simulink model "Atos_Simulink15.3.19"  (R2018b)
settings: Solver=VariableStepAuto  StartTime=0  StopTime=24  FixedStep=1  RelTol=1.0e-3  AbsTol=1.0e-3  EnableMultiTasking=on
libraries: fl_lib x33, nesl_utility x15, SimscapeFluids_lib x2
settings Model: Creator=psytg1  LastModifiedBy=shama
settings SolverCC: AutoScaleAbsTol=off  MaxConsecutiveMinStep=50
settings DataIOCC: LimitDataPoints=on  MaxDataPoints=10000
settings OptimizationCC: LifeSpan=inf
settings DebuggingCC: AllowSymbolicDim=off  LibraryContextMissingDiagnostic=none  SFUnexpectedBacktrackingDiag=warning  SFNoUnconditionalDefaultTransitionDiag=warning  SFExecutionAtInitializationDiag=none
settings SFSimCC: SimUseLocalCustomCode=off
settings RTWCC: GenCodeOnly=on  RTWUseLocalCustomCode=off  TargetLang=C++
settings CodeAppCC: StateflowObjectComments=on
settings GRTTargetCC: TargetLangStandard=C++03 (ISO)  GeneratePreprocessorConditionals=Disable all  MultiInstanceERTCode=on  CodeInterfacePackaging=C++ class
settings ConfigComp: CovMetricSettings=dw  CovHtmlReporting=on  CovSaveCumulativeToWorkspaceVar=on  CovSaveSingleToWorkspaceVar=on  CovExternalEMLEnable=off  CovSFcnEnable=off
settings SimscapeCC: ExplicitSolverDiagnosticOptions=none  SimscapeLogType=all  SimscapeLogDataHistory=10000

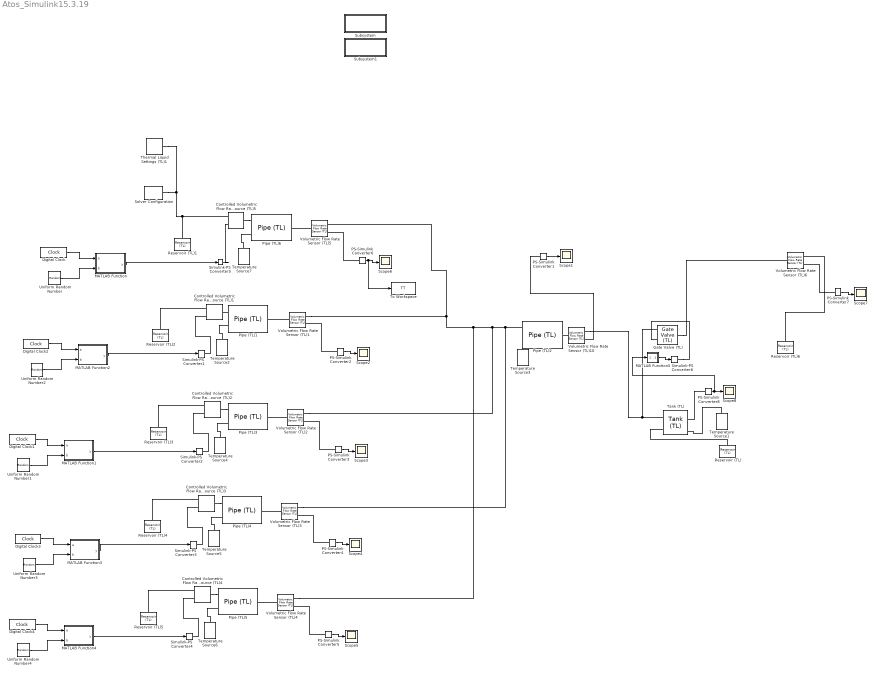
== system Atos_Simulink15.3.19 ==
  Controlled Volumetric Flow Rate Source (TL){1..5} (5 alike) : fl_lib/Thermal Liquid/Sources/Controlled Volumetric Flow Rate Source (TL)  area=3.14 m^2  length=0.1 m  mdot_A_specify=off  mdot_A_priority=None  mdot_A=1 kg/s  mdot_A_nominal_specify=off  mdot_A_nominal_unit=kg/s  mdot_A_nominal_value=1
      settings: SourceProductName=Simscape  SourceProductBaseCode=SS
  Digital Clock{,1..4} (5 alike) : DigitalClock
  Gate Valve (TL) : SimscapeFluids_lib/Thermal Liquid/Valves & Orifices/Flow Control Valves/Gate Valve (TL)  diam_orifice=3 m  x_0=0 m  area_leak=1e-12 m^2  smoothing_factor=1  area=30 m^2  length=1 m  Cd=0.7  Re_c=12  mdot_A_specify=off  mdot_A_priority=None  mdot_A=1 kg/s  mdot_A_nominal_specify=off  mdot_A_nominal_unit=kg/s  mdot_A_nominal_value=1
      settings: SourceProductName=Simscape Fluids  SourceProductBaseCode=SH
  MATLAB Function : MATLAB Function  TreatAsAtomicUnit=on
  MATLAB Function1 : MATLAB Function  TreatAsAtomicUnit=on
  MATLAB Function2 : MATLAB Function  TreatAsAtomicUnit=on
  MATLAB Function3 : MATLAB Function  TreatAsAtomicUnit=on
  MATLAB Function4 : MATLAB Function  TreatAsAtomicUnit=on
  MATLAB Function5 : MATLAB Function  TreatAsAtomicUnit=on
  PS-Simulink Converter{1..8} (8 alike) : nesl_utility/PS-Simulink Converter  PhysicalDomain=network_engine_domain  SubClassName=ps_output  LeftPortType=input  RightPortType=output  PseudoPeriodic=off  Frequencies=[]  Unit=1  AffineConversion=off
  Pipe (TL){1,3..6} (5 alike) : fl_lib/Thermal Liquid/Elements/Pipe (TL)  dynamic_compressibility=1  inertia=0  length=5 m  area=CrossArea m^2  Dh=0.1128 m  length_add=1 m  roughness=15e-6 m  Re_lam=2000  Re_tur=4000  shape_factor=64  Nu_lam=3.66  p0=0.101325 MPa  T0=281.15 K  mdot0=0 kg/s
      settings: SourceProductName=Simscape  SourceProductBaseCode=SS
  Pipe (TL)2 : fl_lib/Thermal Liquid/Elements/Pipe (TL)  dynamic_compressibility=1  inertia=0  length=10 m  area=30 m^2  Dh=0.1128 m  length_add=1 m  roughness=15e-6 m  Re_lam=2000  Re_tur=4000  shape_factor=64  Nu_lam=3.66  p0=0.101325 MPa  T0=281.15 K  mdot0=0 kg/s
      settings: SourceProductName=Simscape  SourceProductBaseCode=SS
  Reservoir (TL) : fl_lib/Thermal Liquid/Elements/Reservoir (TL)  pressure_spec=1  reservoir_pressure=0.101325 MPa  reservoir_temperature=293.15 K  area=3.14 m^2
      settings: SourceProductName=Simscape  SourceProductBaseCode=SS
  Reservoir (TL){1..5} (5 alike) : fl_lib/Thermal Liquid/Elements/Reservoir (TL)  pressure_spec=1  reservoir_pressure=0.101325 MPa  reservoir_temperature=293.15 K  area=0.01 m^2
      settings: SourceProductName=Simscape  SourceProductBaseCode=SS
  Reservoir (TL)6 : fl_lib/Thermal Liquid/Elements/Reservoir (TL)  pressure_spec=1  reservoir_pressure=0.101325 MPa  reservoir_temperature=293.15 K  area=15.7 m^2
      settings: SourceProductName=Simscape  SourceProductBaseCode=SS
  Scope{1..8} (8 alike) : Scope
  Simulink-PS Converter{1..6} (6 alike) : nesl_utility/Simulink-PS Converter  PhysicalDomain=network_engine_domain  SubClassName=ps_input  LeftPortType=input  RightPortType=output  PseudoPeriodic=off  Frequencies=[]  NoiseDistribution=none  NoiseParameters=[]  Unit=1  AffineConversion=off  FilteringAndDerivatives=filter  SimscapeFilterOrder=1  InputFilterTimeConstant=0.001  UdotUserProvided=0
  Solver Configuration : nesl_utility/Solver Configuration  PhysicalDomain=network_engine_domain  SubClassName=solver  LeftPortType=input  RightPortType=generic  Tones=[]  Harmonics=[]  SimulateNoise=off  Profile=off  UseLocalSampling=off  EnableSwitchedLinearOptims=on  FrequencyDomain=off  UseCCode=off  RelTol=0.001  AbsTol=1e-06  MinStep=1e-09  ToWorkspace=off  RevertToSquareIcSolve=off  NumHomotopyIterations=100  PhasorMode=off  PhasorModeNumHarmonics=1  DoDC=off  ResidualTolerance=1e-09  UseLocalSolver=off  LocalSolverChoice=NE_BACKWARD_EULER_ADVANCER  LocalSolverSampleTime=0.001  DoFixedCost=off  MaxNonlinIter=3  MaxModeIter=2  LinearAlgebra=Sparse  EquationFormulation=NE_TIME_EF  DelaysMemoryBudget=1024  AutomaticFiltering=on  FilteringTimeConstant=0.001  PartitionStorageMethod=AS_NEEDED  PartitionMemoryBudget=1024
  Subsystem : Subsystem
      settings: OpenFcn=open_system('simscape')
      mask Display: disp(sprintf('Open Simscape\nLibrary'));
  Subsystem1 : Subsystem
      settings: OpenFcn=|
      | load_system('fl_lib');
      | open_system('fl_lib/Thermal Liquid');
      mask Display: disp(sprintf('Open Thermal Liquid\nLibrary'));
  Tank (TL) : SimscapeFluids_lib/Thermal Liquid/Tanks & Accumulators/Tank (TL)  pressure_spec=1  tank_pressure=0.101325 MPa  max_capacity=10000 m^3  volume_spec=1  tank_area=50 m^2  level_TLU=[0, 3, 5] m  volume_TLU=[0, 4, 6] m^3  inlet_height=1 m  inlet_area=3.14 m^2  g=9.81 m/s^2  level_specify=on  level_priority=High  level=10 m  level_nominal_specify=off  level_nominal_unit=m  level_nominal_value=1  volume_specify=on  volume_priority=None  volume=10 m^3  volume_nominal_specify=off  volume_nominal_unit=m^3  volume_nominal_value=1  mass_specify=on  mass_priority=None  mass=10e+3 kg  mass_nominal_specify=off  mass_nominal_unit=kg  mass_nominal_value=1  T_tank_specify=on  T_tank_priority=High  T_tank=281.15 K  T_tank_nominal_specify=off  T_tank_nominal_unit=K  T_tank_nominal_value=1  inlet_heights_AB=[5, 1] m  inlet_areas_AB=[10, 1] m^2  inlet_heights_ABC=[5, 5, 1] m  inlet_areas_ABC=[10, 10, 1] m^2
      settings: SourceProductName=Simscape Fluids  SourceProductBaseCode=SH
  Temperature Source{1..7} (7 alike) : fl_lib/Thermal/Thermal Sources/Temperature Source  temperature=281.15 K
      settings: SourceProductName=Simscape
  Thermal Liquid Settings (TL)1 : fl_lib/Thermal Liquid/Utilities/Thermal Liquid Settings (TL)  table_dimensions=0  T_TLU=[273.1600 : 10 : 373.16]' K  p_TLU=[0.01, 0.1, 5 : 5 : 50] MPa  p_atm=0.101325 MPa  pT_region_flag=0  T_min=273.16 K  T_max=363.16 K  p_min=0.05 MPa  p_max=50 MPa  T_min_1D=273.16 K  T_max_1D=363.16 K  p_min_1D=0.05 MPa  p_max_1D=50 MPa  pT_validity_TLU=[1, 1, 1, 1, 1, 1, 1, 1, 1, 1, 1, 1; 1, 1, 1, 1, 1, 1, 1, 1, 1, 1, 1, 1; 1, 1, 1, 1, 1, 1, 1, 1, 1, 1, 1, 1; 1, 1, 1, 1, 1, 1, 1, 1, 1, 1, 1, 1; 1, 1, 1, 1, 1, 1, 1, 1, 1, 1, 1, 1; 0, 1, 1, 1, 1, 1, 1, 1, 1, 1, 1, 1; 0, 1, 1, 1, 1, 1, 1, 1, 1, 1, 1, 1; 0, 1, 1, 1, 1, 1, 1, 1, 1, 1, 1, 1; 0, 1, 1, 1, 1, 1, 1, 1, 1, 1, 1, 1; 0, 1, 1, 1, 1, 1, 1, 1, 1, 1, 1, 1; 0, 0, 1, 1, 1, 1, 1, 1, 1, 1, 1, 1]  rho_parameterization_2D=3  rho_parameterization_1D=1  rho_TLU=[999.7973, 999.8431, 1002.3216, 1004.8218, 1007.293, 1009.7358, 1012.1506, 1014.5379, 1016.8979, 1019.2311, 1021.538, 1023.8188; 999.6579, 999.7009, 1002.0303, 1004.382, 1006.7084, 1009.0101, 1011.2874, 1013.5407, 1015.7703, 1017.9766, 1020.1599, 1022.3206; 998.1632, 998.2045, 1000.4375, 1002.6924, 1004.9239, 1007.1324, 1009.3183, 1011.4819, 1013.6236, 1015.7438, 1017.8428, 1019.921; 995.6057, 995.6458, 997.81864, 1000.0128, 1002.1841, 1004.3332, 1006.4603, 1008.566, 1010.6505, 1012.7144, 1014.758, 1016.7815; 992.1724, 992.2119, 994.35133, 996.5113, 998.6484, 1000.7633, 1002.8563, 1004.928, 1006.9788, 1009.009, 1011.0192, 1013.0097; 988.02, 988.0299, 990.15684, 992.3035, 994.4268, 996.5273, 998.6056, 1000.6622, 1002.6976, 1004.7123, 1006.7067, 1008.6813; 983.18, 983.1901, 985.3217, 987.4721, 989.5983, 991.7008, 993.7803, 995.8374, 997.8726, 999.8864, 1001.8795, 1003.8522; 977.75, 977.7583, 979.9094, 982.0783, 984.2216, 986.34, 988.4343, 990.505, 992.5529, 994.5786, 996.5825, 998.5654; 971.77, 971.7836, 973.96734, 976.1678, 978.3409, 980.4876, 982.6087, 984.7049, 986.7768, 988.8254, 990.8511, 992.8545; 965.26, 965.3023, 967.53107, 969.7753, 971.9901, 974.1764, 976.3354, 978.4676, 980.5741, 982.6556, 984.7129, 986.7465; 958.62, 958.6315, 960.627, 962.9267, 965.1944, 967.4314, 969.6387, 971.8173, 973.9681, 976.0921, 978.19, 980.2628] kg/m^3  beta_TLU=[1.9649, 1.9654, 1.9929, 2.0213, 2.0499, 2.0787, 2.1078, 2.1372, 2.1668, 2.1966, 2.2268, 2.2572; 2.0913, 2.0918, 2.1191, 2.1471, 2.1752, 2.2036, 2.2322, 2.261, 2.2899, 2.3191, 2.3485, 2.3781; 2.1786, 2.1791, 2.2067, 2.235, 2.2634, 2.2919, 2.3206, 2.3494, 2.3784, 2.4075, 2.4367, 2.4661; 2.2332, 2.2337, 2.2619, 2.2908, 2.3197, 2.3487, 2.3778, 2.407, 2.4363, 2.4657, 2.4951, 2.5246; 2.26, 2.2605, 2.2895, 2.3191, 2.3487, 2.3784, 2.4081, 2.4378, 2.4675, 2.4973, 2.5272, 2.5571; 2.2638, 2.2638, 2.2936, 2.324, 2.3544, 2.3848, 2.4151, 2.4455, 2.4758, 2.5062, 2.5365, 2.5669; 2.2472, 2.2472, 2.2779, 2.3092, 2.3403, 2.3715, 2.4025, 2.4336, 2.4646, 2.4955, 2.5264, 2.5573; 2.214, 2.214, 2.2455, 2.2776, 2.3096, 2.3415, 2.3733, 2.405, 2.4367, 2.4683, 2.4998, 2.5313; 2.1668, 2.1668, 2.1992, 2.2321, 2.2649, 2.2976, 2.3301, 2.3626, 2.3949, 2.4272, 2.4593, 2.4914; 2.1081, 2.1081, 2.1413, 2.175, 2.2086, 2.2421, 2.2754, 2.3085, 2.3415, 2.3744, 2.4072, 2.4399; 2.0494, 2.0494, 2.0739, 2.1084, 2.1428, 2.177, 2.211, 2.2449, 2.2786, 2.3121, 2.3455, 2.3788] GPa  alpha_TLU=1e-4 * [-.679, -.676, -.49, -.307, -.13, .041, .206, .365, .519, .668, .811, .949; .878, .881, .998, 1.114, 1.227, 1.337, 1.445, 1.549, 1.651, 1.75, 1.846, 1.939; 2.068, 2.069, 2.141, 2.213, 2.283, 2.352, 2.42, 2.486, 2.551, 2.614, 2.676, 2.736; 3.034, 3.035, 3.074, 3.113, 3.152, 3.191, 3.229, 3.267, 3.305, 3.341, 3.377, 3.413; 3.855, 3.856, 3.87, 3.884, 3.899, 3.914, 3.93, 3.946, 3.961, 3.977, 3.993, 4.009; 4.578, 4.578, 4.572, 4.566, 4.562, 4.558, 4.555, 4.552, 4.55, 4.549, 4.548, 4.547; 5.233, 5.233, 5.209, 5.186, 5.165, 5.144, 5.125, 5.107, 5.09, 5.074, 5.059, 5.045; 5.84, 5.84, 5.801, 5.762, 5.725, 5.691, 5.657, 5.625, 5.595, 5.566, 5.538, 5.512; 6.414, 6.414, 6.36, 6.307, 6.256, 6.208, 6.161, 6.117, 6.074, 6.033, 5.994, 5.956; 6.967, 6.967, 6.898, 6.831, 6.766, 6.705, 6.646, 6.589, 6.535, 6.482, 6.432, 6.384; 7.519, 7.519, 7.423, 7.342, 7.264, 7.189, 7.118, 7.049, 6.983, 6.92, 6.859, 6.8] 1/K  rho_TLU_2=[999.7973, 999.8431, 1002.3216, 1004.8218, 1007.293, 1009.7358, 1012.1506, 1014.5379, 1016.8979, 1019.2311, 1021.538, 1023.8188; 999.6579, 999.7009, 1002.0303, 1004.382, 1006.7084, 1009.0101, 1011.2874, 1013.5407, 1015.7703, 1017.9766, 1020.1599, 1022.3206; 998.1632, 998.2045, 1000.4375, 1002.6924, 1004.9239, 1007.1324, 1009.3183, 1011.4819, 1013.6236, 1015.7438, 1017.8428, 1019.921; 995.6057, 995.6458, 997.81864, 1000.0128, 1002.1841, 1004.3332, 1006.4603, 1008.566, 1010.6505, 1012.7144, 1014.758, 1016.7815; 992.1724, 992.2119, 994.35133, 996.5113, 998.6484, 1000.7633, 1002.8563, 1004.928, 1006.9788, 1009.009, 1011.0192, 1013.0097; 988.02, 988.0299, 990.15684, 992.3035, 994.4268, 996.5273, 998.6056, 1000.6622, 1002.6976, 1004.7123, 1006.7067, 1008.6813; 983.18, 983.1901, 985.3217, 987.4721, 989.5983, 991.7008, 993.7803, 995.8374, 997.8726, 999.8864, 1001.8795, 1003.8522; 977.75, 977.7583, 979.9094, 982.0783, 984.2216, 986.34, 988.4343, 990.505, 992.5529, 994.5786, 996.5825, 998.5654; 971.77, 971.7836, 973.96734, 976.1678, 978.3409, 980.4876, 982.6087, 984.7049, 986.7768, 988.8254, 990.8511, 992.8545; 965.26, 965.3023, 967.53107, 969.7753, 971.9901, 974.1764, 976.3354, 978.4676, 980.5741, 982.6556, 984.7129, 986.7465; 958.62, 958.6315, 960.627, 962.9267, 965.1944, 967.4314, 969.6387, 971.8173, 973.9681, 976.0921, 978.19, 980.2628] kg/m^3  rho_ref_3=978.19 kg/m^3  T_ref_3=293.16 K  p_ref_3=0.101325 MPa  beta_const_3=2.1791 GPa  alpha_const_3=2.0691e-4 1/K  rho_TLU_4=[999.84; 999.7; 998.2; 995.65; 992.21; 988.03; 983.19; 977.76; 971.78; 965.3; 958.8] kg/m^3  beta_const_4=2.1791 GPa  p_ref_4=0.101325 MPa  rho_ref_5=998.21 kg/m^3  T_ref_5=293.16 K  p_ref_5=0.101325 MPa  beta_const_5=2.1791 GPa  alpha_const_5=2.0691e-4 1/K  u_parameterization_2D=1  u_parameterization_1D=1  u_TLU=[.0002, .0018, .086, .1588, .219, .267, .3034, .3288, .3436, .3483, .3435, .3294; 42.062, 42.06, 41.935, 41.804, 41.668, 41.527, 41.382, 41.233, 41.081, 40.924, 40.763, 40.599; 83.953, 83.948, 83.651, 83.349, 83.049, 82.749, 82.451, 82.153, 81.856, 81.56, 81.265, 80.971; 125.77, 125.76, 125.31, 124.86, 124.41, 123.97, 123.53, 123.1, 122.68, 122.25, 121.84, 121.42; 167.57, 167.56, 166.96, 166.37, 165.79, 165.21, 164.65, 164.09, 163.54, 163, 162.46, 161.94; 209.36, 209.36, 208.63, 207.9, 207.19, 206.48, 205.79, 205.11, 204.45, 203.79, 203.14, 202.5; 251.19, 251.19, 250.33, 249.47, 248.62, 247.79, 246.98, 246.18, 245.39, 244.62, 243.86, 243.12; 293.06, 293.06, 292.07, 291.07, 290.1, 289.14, 288.2, 287.28, 286.38, 285.49, 284.62, 283.77; 334.99, 334.99, 333.86, 332.73, 331.63, 330.54, 329.48, 328.44, 327.41, 326.41, 325.43, 324.46; 377, 377, 375.73, 374.46, 373.22, 372, 370.81, 369.64, 368.5, 367.38, 366.27, 365.19; 419.01, 419.01, 417.69, 416.27, 414.89, 413.54, 412.21, 410.91, 409.64, 408.4, 407.17, 405.98] kJ/kg  cp_TLU=[4.2199, 4.2194, 4.1957, 4.1726, 4.1508, 4.13, 4.1103, 4.0916, 4.0738, 4.0569, 4.0408, 4.0254; 4.1955, 4.1951, 4.1769, 4.1592, 4.1422, 4.1259, 4.1103, 4.0954, 4.0812, 4.0676, 4.0545, 4.0421; 4.1843, 4.184, 4.169, 4.1543, 4.1401, 4.1264, 4.1133, 4.1007, 4.0885, 4.0768, 4.0656, 4.0548; 4.1801, 4.1798, 4.1667, 4.1538, 4.1413, 4.1293, 4.1177, 4.1064, 4.0956, 4.0851, 4.075, 4.0653; 4.1796, 4.1794, 4.1675, 4.1558, 4.1444, 4.1334, 4.1227, 4.1123, 4.1023, 4.0926, 4.0832, 4.0741; 4.1813, 4.1813, 4.1702, 4.1592, 4.1484, 4.138, 4.1279, 4.1181, 4.1086, 4.0993, 4.0903, 4.0816; 4.185, 4.185, 4.1742, 4.1636, 4.1532, 4.1432, 4.1334, 4.1239, 4.1146, 4.1056, 4.0969, 4.0884; 4.1901, 4.1901, 4.1795, 4.169, 4.1588, 4.1489, 4.1393, 4.1299, 4.1207, 4.1118, 4.1032, 4.0947; 4.1968, 4.1968, 4.1862, 4.1757, 4.1655, 4.1555, 4.1458, 4.1364, 4.1273, 4.1183, 4.1096, 4.1012; 4.2052, 4.2052, 4.1944, 4.1837, 4.1733, 4.1632, 4.1534, 4.1438, 4.1345, 4.1255, 4.1166, 4.108; 4.2136, 4.2136, 4.2045, 4.1935, 4.1828, 4.1724, 4.1623, 4.1524, 4.1429, 4.1335, 4.1245, 4.1157] kJ/kg/K  u_TLU_2=[.0002, .0018, .086, .1588, .219, .267, .3034, .3288, .3436, .3483, .3435, .3294; 42.062, 42.06, 41.935, 41.804, 41.668, 41.527, 41.382, 41.233, 41.081, 40.924, 40.763, 40.599; 83.953, 83.948, 83.651, 83.349, 83.049, 82.749, 82.451, 82.153, 81.856, 81.56, 81.265, 80.971; 125.77, 125.76, 125.31, 124.86, 124.41, 123.97, 123.53, 123.1, 122.68, 122.25, 121.84, 121.42; 167.57, 167.56, 166.96, 166.37, 165.79, 165.21, 164.65, 164.09, 163.54, 163, 162.46, 161.94; 209.36, 209.36, 208.63, 207.9, 207.19, 206.48, 205.79, 205.11, 204.45, 203.79, 203.14, 202.5; 251.19, 251.19, 250.33, 249.47, 248.62, 247.79, 246.98, 246.18, 245.39, 244.62, 243.86, 243.12; 293.06, 293.06, 292.07, 291.07, 290.1, 289.14, 288.2, 287.28, 286.38, 285.49, 284.62, 283.77; 334.99, 334.99, 333.86, 332.73, 331.63, 330.54, 329.48, 328.44, 327.41, 326.41, 325.43, 324.46; 377, 377, 375.73, 374.46, 373.22, 372, 370.81, 369.64, 368.5, 367.38, 366.27, 365.19; 419.01, 419.01, 417.69, 416.27, 414.89, 413.54, 412.21, 410.91, 409.64, 408.4, 407.17, 405.98] kJ/kg  cp_TLU_3=[4.2199, 4.2194, 4.1957, 4.1726, 4.1508, 4.13, 4.1103, 4.0916, 4.0738, 4.0569, 4.0408, 4.0254; 4.1955, 4.1951, 4.1769, 4.1592, 4.1422, 4.1259, 4.1103, 4.0954, 4.0812, 4.0676, 4.0545, 4.0421; 4.1843, 4.184, 4.169, 4.1543, 4.1401, 4.1264, 4.1133, 4.1007, 4.0885, 4.0768, 4.0656, 4.0548; 4.1801, 4.1798, 4.1667, 4.1538, 4.1413, 4.1293, 4.1177, 4.1064, 4.0956, 4.0851, 4.075, 4.0653; 4.1796, 4.1794, 4.1675, 4.1558, 4.1444, 4.1334, 4.1227, 4.1123, 4.1023, 4.0926, 4.0832, 4.0741; 4.1813, 4.1813, 4.1702, 4.1592, 4.1484, 4.138, 4.1279, 4.1181, 4.1086, 4.0993, 4.0903, 4.0816; 4.185, 4.185, 4.1742, 4.1636, 4.1532, 4.1432, 4.1334, 4.1239, 4.1146, 4.1056, 4.0969, 4.0884; 4.1901, 4.1901, 4.1795, 4.169, 4.1588, 4.1489, 4.1393, 4.1299, 4.1207, 4.1118, 4.1032, 4.0947; 4.1968, 4.1968, 4.1862, 4.1757, 4.1655, 4.1555, 4.1458, 4.1364, 4.1273, 4.1183, 4.1096, 4.1012; 4.2052, 4.2052, 4.1944, 4.1837, 4.1733, 4.1632, 4.1534, 4.1438, 4.1345, 4.1255, 4.1166, 4.108; 4.2136, 4.2136, 4.2045, 4.1935, 4.1828, 4.1724, 4.1623, 4.1524, 4.1429, 4.1335, 4.1245, 4.1157] kJ/kg/K  u_TLU_4=[.0018; 42.06; 83.948; 125.76; 167.56; 209.36; 251.19; 293.06; 334.99; 377; 418.01] kJ/kg  cp_TLU_5=[4.2199; 4.1955; 4.1843; 4.1801; 4.1796; 4.1813; 4.185; 4.1901; 4.1968; 4.2052; 4.2136] kJ/kg/K  nu_TLU=[1.7917, 1.7914, 1.7763, 1.7615, 1.7473, 1.7338, 1.7208, 1.7085, 1.6967, 1.6854, 1.6747, 1.6645; 1.3061, 1.3059, 1.2986, 1.2914, 1.2845, 1.2779, 1.2716, 1.2656, 1.2598, 1.2543, 1.2491, 1.2441; 1.0032, 1.0032, .9995, .9959, .9924, .9891, .9859, .9829, .9801, .9774, .9748, .9724; .8006, .8005, .7987, .797, .7953, .7937, .7922, .7908, .7894, .7881, .787, .7859; .6577, .6577, .657, .6562, .6555, .6548, .6543, .6537, .6532, .6528, .6523, .652; .553, .553, .5529, .5527, .5526, .5525, .5524, .5524, .5524, .5524, .5524, .5525; .4739, .4739, .4741, .4743, .4745, .4747, .475, .4753, .4755, .4758, .4762, .4765; .4127, .4127, .4131, .4135, .4139, .4143, .4148, .4152, .4157, .4162, .4167, .4172; .3643, .3643, .3648, .3654, .3659, .3665, .367, .3676, .3682, .3688, .3694, .37; .3254, .3254, .3261, .3267, .3273, .328, .3286, .3293, .3299, .3306, .3312, .3319; .2866, .2866, .2945, .2952, .2959, .2965, .2972, .2979, .2986, .2993, .3, .3007] mm^2/s  nu_TLU_2=[1.7917; 1.3061; 1.0032; .8006; .6577; .553; .4739; .4127; .3643; .3254; .2866] mm^2/s  k_TLU=[561.04, 561.09, 563.8, 566.56, 569.32, 572.08, 574.82, 577.54, 580.24, 582.92, 585.57, 588.18; 580.02, 580.07, 582.45, 584.88, 587.32, 589.75, 592.18, 594.61, 597.02, 599.42, 601.8, 604.16; 598.44, 598.48, 600.73, 603.03, 605.33, 607.64, 609.94, 612.24, 614.54, 616.82, 619.1, 621.36; 615.48, 615.52, 617.73, 620, 622.26, 624.54, 626.81, 629.07, 631.34, 633.6, 635.85, 638.09; 630.6, 630.64, 632.87, 635.15, 637.44, 639.72, 642.01, 644.29, 646.57, 648.84, 651.11, 653.36; 643.61, 643.61, 645.88, 648.21, 650.53, 652.86, 655.18, 657.51, 659.82, 662.14, 664.44, 666.74; 654.39, 654.39, 656.73, 659.12, 661.5, 663.89, 666.27, 668.65, 671.02, 673.38, 675.74, 678.09; 663.13, 663.13, 665.54, 668, 670.46, 672.91, 675.36, 677.8, 680.24, 682.67, 685.09, 687.5; 670.02, 670.02, 672.51, 675.05, 677.59, 680.12, 682.64, 685.16, 687.67, 690.17, 692.66, 695.14; 675.27, 675.27, 677.85, 680.48, 683.11, 685.73, 688.34, 690.94, 693.53, 696.11, 698.68, 701.24; 680.52, 680.52, 681.77, 684.5, 687.22, 689.94, 692.64, 695.34, 698.02, 700.69, 703.35, 706] mW/m/K  k_TLU_2=[561.04; 580.02; 598.44; 615.48; 630.6; 643.61; 654.39; 663.13; 670.02; 675.27; 680.52] mW/m/K
      settings: SourceProductName=Simscape  SourceProductBaseCode=SS
  To Workspace : ToWorkspace  VariableName=TT  SaveFormat=Timeseries  SampleTime=-1
  Uniform Random Number{,1..4} (5 alike) : UniformRandomNumber  Minimum=4  Maximum=6  SampleTime=1  VectorParams1D=off
  Volumetric Flow Rate Sensor (TL){1..6,10} (7 alike) : fl_lib/Thermal Liquid/Sensors/Volumetric Flow Rate Sensor (TL)
      settings: SourceProductName=Simscape  SourceProductBaseCode=SS  LogSimulationData=on
  wires:
  PS-Simulink Converter1/1 -> Scope1/1
  PS-Simulink Converter2/1 -> Scope2/1
  PS-Simulink Converter3/1 -> Scope3/1
  PS-Simulink Converter4/1 -> Scope4/1
  PS-Simulink Converter5/1 -> Scope5/1
  PS-Simulink Converter6/1 -> To Workspace/1, Scope6/1
  PS-Simulink Converter8/1 -> MATLAB Function5/1(u), Scope8/1
  Digital Clock/1 -> MATLAB Function/1(a)
  MATLAB Function/1(y) -> Simulink-PS Converter5/1
  Uniform Random Number/1 -> MATLAB Function/2(b)
  MATLAB Function1/1(y) -> Simulink-PS Converter2/1
  Digital Clock1/1 -> MATLAB Function1/1(a)
  Uniform Random Number1/1 -> MATLAB Function1/2(b)
  MATLAB Function2/1(y) -> Simulink-PS Converter1/1
  Digital Clock2/1 -> MATLAB Function2/1(a)
  Uniform Random Number2/1 -> MATLAB Function2/2(b)
  MATLAB Function3/1(y) -> Simulink-PS Converter3/1
  Digital Clock3/1 -> MATLAB Function3/1(a)
  Uniform Random Number3/1 -> MATLAB Function3/2(b)
  MATLAB Function4/1(y) -> Simulink-PS Converter4/1
  Digital Clock4/1 -> MATLAB Function4/1(a)
  Uniform Random Number4/1 -> MATLAB Function4/2(b)
  MATLAB Function5/1(y) -> Simulink-PS Converter6/1
  PS-Simulink Converter7/1 -> Scope7/1
  connections:
  Reservoir (TL)2/LConn1 -- Controlled Volumetric Flow Rate Source (TL)1/LConn1
  Temperature Source2/LConn1 -- Pipe (TL)1/LConn2
  Controlled Volumetric Flow Rate Source (TL)1/RConn1 -- Pipe (TL)1/LConn1
  Volumetric Flow Rate Sensor (TL)1/LConn1 -- Pipe (TL)1/RConn1
  Temperature Source3/LConn1 -- Pipe (TL)2/LConn2
  Volumetric Flow Rate Sensor (TL)10/LConn1 -- Pipe (TL)2/RConn1
  PS-Simulink Converter1/LConn1 -- Volumetric Flow Rate Sensor (TL)10/RConn2
  Simulink-PS Converter1/RConn1 -- Controlled Volumetric Flow Rate Source (TL)1/LConn2
  PS-Simulink Converter2/LConn1 -- Volumetric Flow Rate Sensor (TL)1/RConn2
  Simulink-PS Converter2/RConn1 -- Controlled Volumetric Flow Rate Source (TL)2/LConn2
  Temperature Source4/LConn1 -- Pipe (TL)3/LConn2
  Volumetric Flow Rate Sensor (TL)2/LConn1 -- Pipe (TL)3/RConn1
  PS-Simulink Converter3/LConn1 -- Volumetric Flow Rate Sensor (TL)2/RConn2
  Controlled Volumetric Flow Rate Source (TL)2/RConn1 -- Pipe (TL)3/LConn1
  Reservoir (TL)3/LConn1 -- Controlled Volumetric Flow Rate Source (TL)2/LConn1
  Simulink-PS Converter3/RConn1 -- Controlled Volumetric Flow Rate Source (TL)3/LConn2
  Temperature Source5/LConn1 -- Pipe (TL)4/LConn2
  Volumetric Flow Rate Sensor (TL)3/LConn1 -- Pipe (TL)4/RConn1
  PS-Simulink Converter4/LConn1 -- Volumetric Flow Rate Sensor (TL)3/RConn2
  Controlled Volumetric Flow Rate Source (TL)3/RConn1 -- Pipe (TL)4/LConn1
  Reservoir (TL)4/LConn1 -- Controlled Volumetric Flow Rate Source (TL)3/LConn1
  Simulink-PS Converter4/RConn1 -- Controlled Volumetric Flow Rate Source (TL)4/LConn2
  Temperature Source6/LConn1 -- Pipe (TL)5/LConn2
  Volumetric Flow Rate Sensor (TL)4/LConn1 -- Pipe (TL)5/RConn1
  PS-Simulink Converter5/LConn1 -- Volumetric Flow Rate Sensor (TL)4/RConn2
  Controlled Volumetric Flow Rate Source (TL)4/RConn1 -- Pipe (TL)5/LConn1
  Reservoir (TL)5/LConn1 -- Controlled Volumetric Flow Rate Source (TL)4/LConn1
  Solver Configuration/RConn1 -- Thermal Liquid Settings (TL)1/RConn1 -- Controlled Volumetric Flow Rate Source (TL)5/LConn1 -- Reservoir (TL)1/LConn1
  Temperature Source7/LConn1 -- Pipe (TL)6/LConn2
  Volumetric Flow Rate Sensor (TL)5/LConn1 -- Pipe (TL)6/RConn1
  Controlled Volumetric Flow Rate Source (TL)5/RConn1 -- Pipe (TL)6/LConn1
  PS-Simulink Converter6/LConn1 -- Volumetric Flow Rate Sensor (TL)5/RConn2
  Temperature Source1/LConn1 -- Tank (TL)/RConn4
  Simulink-PS Converter5/RConn1 -- Controlled Volumetric Flow Rate Source (TL)5/LConn2
  Volumetric Flow Rate Sensor (TL)10/RConn1 -- Tank (TL)/LConn1 -- Gate Valve (TL)/LConn1
  PS-Simulink Converter8/LConn1 -- Tank (TL)/RConn2
  Volumetric Flow Rate Sensor (TL)1/RConn1 -- Volumetric Flow Rate Sensor (TL)4/RConn1 -- Volumetric Flow Rate Sensor (TL)3/RConn1 -- Pipe (TL)2/LConn1 -- Volumetric Flow Rate Sensor (TL)2/RConn1 -- Volumetric Flow Rate Sensor (TL)5/RConn1
  Reservoir (TL)6/LConn1 -- Volumetric Flow Rate Sensor (TL)6/RConn1
  Simulink-PS Converter6/RConn1 -- Gate Valve (TL)/LConn2
  PS-Simulink Converter7/LConn1 -- Volumetric Flow Rate Sensor (TL)6/RConn2
  Gate Valve (TL)/RConn1 -- Volumetric Flow Rate Sensor (TL)6/LConn1
  Reservoir (TL)/LConn1 -- Tank (TL)/LConn2

== system Atos_Simulink15.3.19/Subsystem ==

== system Atos_Simulink15.3.19/Subsystem1 ==

== matlab function Atos_Simulink15.3.19/MATLAB Function1 ==
  data: y output; a input; b input
function y  = fcn(a , b)

if a >=0 && a <= 6 
    y = b*2;
elseif a > 6 && a <= 11
    y = b * 5 ;
elseif a > 11 && a <= 17
    y= b * 2 ;
elseif a > 17 && a <= 20
    y = b * 5 ;
elseif a> 20 && a <= 24
    y = b * 3 ;
else
    y= 30;
end

== matlab function Atos_Simulink15.3.19/MATLAB Function ==
  data: y output; a input; b input
function y  = fcn(a , b)

if a >=0 && a <= 6 
    y = b*2;
elseif a > 6 && a <= 11
    y = b * 5 ;
elseif a > 11 && a <= 17
    y= b * 2 ;
elseif a > 17 && a <= 20
    y = b * 5 ;
elseif a> 20 && a <= 24
    y = b * 3 ;
else
    y= 30;
end

== matlab function Atos_Simulink15.3.19/MATLAB Function2 ==
  data: y output; a input; b input
function y  = fcn(a , b)

if a >=0 && a <= 6 
    y = b*2;
elseif a > 6 && a <= 11
    y = b * 5 ;
elseif a > 11 && a <= 17
    y= b * 2 ;
elseif a > 17 && a <= 20
    y = b * 5 ;
elseif a> 20 && a <= 24
    y = b * 3 ;
else
    y= 30;
end

== matlab function Atos_Simulink15.3.19/MATLAB Function3 ==
  data: y output; a input; b input
function y  = fcn(a , b)

if a >=0 && a <= 6 
    y = b*2;
elseif a > 6 && a <= 11
    y = b * 5 ;
elseif a > 11 && a <= 17
    y= b * 2 ;
elseif a > 17 && a <= 20
    y = b * 5 ;
elseif a> 20 && a <= 24
    y = b * 3 ;
else
    y= 30;
end

== matlab function Atos_Simulink15.3.19/MATLAB Function4 ==
  data: y output; a input; b input
function y  = fcn(a , b)

if a >=0 && a <= 6 
    y = b*2;
elseif a > 6 && a <= 11
    y = b * 5 ;
elseif a > 11 && a <= 17
    y= b * 2 ;
elseif a > 17 && a <= 20
    y = b * 5 ;
elseif a> 20 && a <= 24
    y = b * 3 ;
else
    y= 30;
end

== matlab function Atos_Simulink15.3.19/MATLAB Function5 ==
  data: u input; y output
function y = fcn(u)

if u >= 30
    y = 6 ;
elseif u <= 10
    y = 0 ;
else
    y = 0 ;
end
